simulink model "VehicleModel_V3"  (R2021b)
settings: Solver=FixedStepAuto  StartTime=0.0  StopTime=4000  FixedStep=Max_StepSize  RelTol=1e-3
InitFcn:
  | addpath('./Include')
  | Vehicle_Parameters
undefined symbols (not defined in the file): Airpressure, drag_coeff, front_area, Gravity, Incline, Ion, Irradiance, Lithium, NextCoordDistance, Temperature, Volume
libraries: spsPVArrayLib x10, spsSeriesRLCBranchLib x10, fl_lib x10, spsCurrentMeasurementLib x7, nesl_utility x6, sdl_lib x5, spsVoltageMeasurementLib x4, spsIGBTDiodeLib x3, spsPWMGeneratorDCDCLib x3, slpidlib x1, spsGroundLib x1, spsBatteryLib x1
settings Model: SimulationMode=accelerator  Creator=Zubim  LastModifiedBy=Zubim
settings SolverCC: MaxConsecutiveZCs=1  ZeroCrossAlgorithm=Adaptive
settings DataIOCC: SaveState=on
settings OptimizationCC: SimCompilerOptimization=on
settings DebuggingCC: StringTruncationChecking=none  IgnoredZcDiagnostic=none  MultiTaskCondExecSysMsg=none  MultiTaskRateTransMsg=warning  TasksWithSamePriorityMsg=none  SigSpecEnsureSampleTimeMsg=none  IntegerOverflowMsg=none  UnknownTsInhSupMsg=none  IntegerSaturationMsg=none
settings SFSimCC: SimCtrlC=off

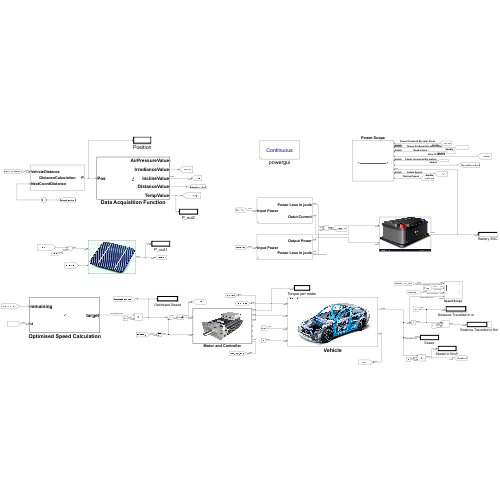
[thumbnail: Simulink's stored preview of the top-level diagram]
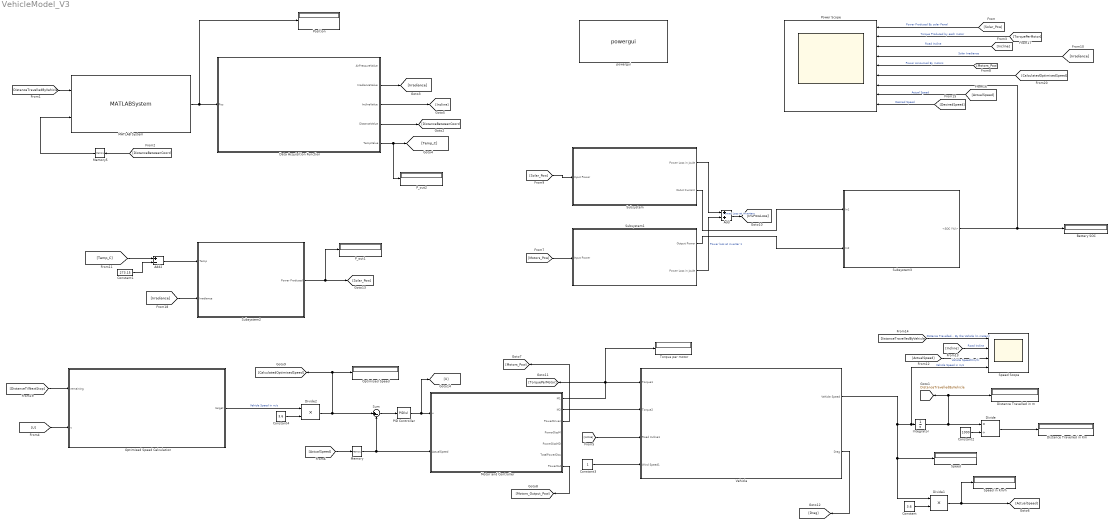
== system VehicleModel_V3 ==
  Add : Sum
  Add2 : Sum  Inputs=+-
  Battery SOC : Display
  Constant : Constant  Value=3.6
  Constant1 : Constant  Value=273.15
  Constant2 : Constant  Value=1000
  Constant3 : Constant
  Constant4 : Constant  Value=3.6
  Data Acquisition Function : MATLAB Function  TreatAsAtomicUnit=on
  Distance Travelled in Km : Display
  Distance Travelled in m : Display
  Divide : Product  Inputs=*/
  Divide1 : Product  Inputs=**
  Divide2 : Product  Inputs=**
  Integrator : Integrator
  MATLAB System : MATLABSystem  System=DistanceCalculation  SimulateUsing=Code generation
      mask Type: DistanceCalculation
      mask Display:
      | disp('DistanceCalculation');
      | port_label('input',1,'VehicleDistance');
      | port_label('input',2,'NextCoordDistance');
      | port_label('output',1,'P');
  Memory : Memory
  Memory5 : Memory  InheritSampleTime=on  LinearizeAsDelay=on
  Motor and Controller : MATLAB Function  TreatAsAtomicUnit=on
  Optimised Speed : Display
  Optimised Speed Calculation : MATLAB Function  TreatAsAtomicUnit=on
  PID Controller : slpidlib/PID Controller  Controller=PID  Form=Parallel  TimeDomain=Continuous-time  UseExternalTs=off  SampleTime=-1  IntegratorMethod=Forward Euler  FilterMethod=Forward Euler  ControllerParametersSource=internal  P=7.5E-1  I=15E-5  D=1.15E-1  UseFilter=on  N=1  TunerSelectOption=Transfer Function Based (PID Tuner App)  InitialConditionSource=internal  InitialConditionForIntegrator=0  InitialConditionForFilter=0  DifferentiatorICPrevScaledInput=0  ExternalReset=none  TrackingMode=off  Kt=1  LimitOutput=on  SatLimitsSource=internal  UpperSaturationLimit=1  LowerSaturationLimit=-0.2  LinearizeAsGain=on  AntiWindupMode=none  Kb=1  POutMin=[]  POutMax=[]  IOutMin=[]  IOutMax=[]  DOutMin=[]  DOutMax=[]  NOutMin=[]  NOutMax=[]  SumOutDataTypeStr=double  SumOutMin=[]  SumOutMax=[]  SaturationOutDataTypeStr=double  SaturationOutMin=[]  SaturationOutMax=[]  PParamMin=[]  PParamMax=[]  IParamMin=[]  IParamMax=[]  DParamMin=[]  DParamMax=[]  NParamMin=[]  NParamMax=[]  KbParamMin=[]  KbParamMax=[]  KtParamMin=[]  KtParamMax=[]  KbOutMin=[]  KbOutMax=[]  KtOutMin=[]  KtOutMax=[]  IntegratorOutMin=[]  IntegratorOutMax=[]  FilterOutMin=[]  FilterOutMax=[]  SumI1OutMin=[]  SumI1OutMax=[]  SumI2OutMin=[]  SumI2OutMax=[]  SumI3OutMin=[]  SumI3OutMax=[]  SumI4OutMin=[]  SumI4OutMax=[]  SumDOutMin=[]  SumDOutMax=[]  DifferentiatorOutMin=[]  DifferentiatorOutMax=[]  FilterDiffOutCoefMin=[]  FilterDiffOutCoefMax=[]  ReciprocalOutMin=[]  ReciprocalOutMax=[]  SumDenOutMin=[]  SumDenOutMax=[]  SumNumOutMin=[]  SumNumOutMax=[]  DivideOutMin=[]  DivideOutMax=[]  UdiffTsProdOutMin=[]  UdiffTsProdOutMax=[]  NTsProdOutMin=[]  NTsProdOutMax=[]  UintegralTsProdOutMin=[]  UintegralTsProdOutMax=[]  UngainTsProdOutMin=[]  UngainTsProdOutMax=[]  IntegratorContinuousStateAttributes=''  IntegratorStateMustResolveToSignalObject=off  IntegratorRTWStateStorageClass=Auto  FilterContinuousStateAttributes=''  FilterStateMustResolveToSignalObject=off  FilterRTWStateStorageClass=Auto  ParallelPVariant=InternalParameters  IdealPVariant=Disabled  IVariant=InternalParameters  DVariant=InternalParameters  IntegratorVariant=Continuous  SatVariant=Enabled  AWVariant=Passthrough  PCopyVariant=Disabled  TRVariant=Disabled  FdbkBlocksVariant=Forward  IdealPFdbkVariant=Disabled  SatFdbkVariant=Disabled  DerivativeFilterVariant=ContFilter  NVariant=InternalParameters  NCopyVariant=Disabled  FilterICVariant=InternalICsFilter  IntegratorICVariant=InternalICs  ExternalResetVariant=Disabled  TRSumVariant=Passthrough  SumFdbkVariant=Disabled  SumVariant=Sum_PID  TsampFilterVariant=InternalTs  TsampNgainVariant=Passthrough  TsampIntegralVariant=Passthrough  ExternalSaturationOutDataTypeStr=Inherit: Same as second input
  P_out1 : Display
  P_out2 : Display
  Position : Display
  Power Scope : Scope  NumInputPorts=9
  Speed : Display
  Speed Scope : Scope  NumInputPorts=4
  Speed in Km/h : Display
  Subsystem : Subsystem  mask{Inv_Efficiency=0.99}
      mask prompts: Inv_Efficiency "Efficiency (value between  0 and 1)"
  Subsystem1 : Subsystem  mask{Inv_Efficiency=0.95}
      mask prompts: Inv_Efficiency "Efficiency (value between  0 and 1)"
  Subsystem2 : Subsystem
      mask Display: image('D:\Vehicle Model\Images\Solar_cell.png'); % Use "Edit Image" on toolstrip to change.
  Subsystem3 : Subsystem
      mask Display: image('D:\Vehicle Model\Images\Battery.jpg'); % Use "Edit Image" on toolstrip to change.
  Sum : Sum  Inputs=|+-
  Torque per motor : Display
  Vehicle : Subsystem
      mask Display: image('D:\3rd Year\Group Project\Vehicle Model Matlab\Vehicle.jpg'); % Use "Edit Image" on toolstrip to change.
  powergui : spspowerguiLib/powergui  Priority=1  SimulationMode=Continuous  SampleTime=1  frequency=60  Iterations=50  frequencyindice=0  Pbase=100e6  ErrMax=1e-4  UnitsV=kV  UnitsW=MW  buscounter=0  FunctionMessages=off  echomessages=off  EnableUseOfTLC=off  CurrentSourceSwitches=off  DisableSnubberDevices=off  DisableRonSwitches=off  DisableVfSwitches=off  DisplayEquations=off  AutomaticDiscreteSolvers=off  SolverType=Tustin/Backward Euler (TBE)  Interpol=off  ExternalGateDelay=off  methode=off  Ts=100  x0status=blocks  SPID=on  SwTol=0  HookPort=off  NonlinearTolerance=1e-4  nMaxIteration=100  ContinueOnMaxIteration=off  RestoreLinks=warning  ResistiveCurrentMeasurement=off  Frange=[0:2:500]  Ylog=off  Xlog=on  ShowGrid=off  save=off  variable=ZData  structure=0  ZoomFFT=off  StartTime=0.0  cycles=1  DisplayStyle=1  fundamental=60  FreqAxis=off  MaxFrequency=1000  frequencyindicesteady=1  RmsSteady=1  display=off
  tag scope: DistanceTravelledByVehicle=global
  wires:
  Subsystem/1(" Power Loss in joule") -> Add/1
  Vehicle/1(Vehicle Speed) -> Speed Scope/4, Integrator/1, Speed/1, Divide1/1  "Vehicle Speed in m/s"
  [DistanceTravelledByVehicle] -> MATLAB System/1
  [DistanceBetweenCoord] -> Memory5/1
  Memory5/1 -> MATLAB System/2
  Constant2/1 -> Divide/2
  Divide/1 -> Distance Travelled in Km/1
  [Incline] -> Vehicle/3(Road Incline1)
  [Solar_Pow] -> Subsystem/1(Input Power)
  MATLAB System/1 -> Position/1, Data Acquisition Function/1(Pos)
  Data Acquisition Function/4(DistanceValue) -> [DistanceBetweenCoord]
  Data Acquisition Function/2(IrradianceValue) -> [Irradiance]
  Data Acquisition Function/5(TempValue) -> P_out2/1, [Temp_C]
  Data Acquisition Function/3(InclineValue) -> [Incline]
  Sum/1 -> PID Controller/1
  PID Controller/1 -> [U], Motor and Controller/1(u)
  [ActualSpeed] -> Memory/1
  [Motors_Pow] -> Power Scope/5  "Power consumed By motors"
  [Irradiance] -> Power Scope/4  "Solar Irradiance"
  Memory/1 -> Sum/2, Motor and Controller/2(ActualSpeed)
  Motor and Controller/2(M2) -> Vehicle/2(Torque2)
  Motor and Controller/1(M1) -> [TorquePerMotor], Torque per motor/1, Vehicle/1(Torque1)
  Constant3/1 -> Vehicle/4(Wind Speed1)
  Motor and Controller/3(PowerDriven) -> [Motors_Pow]
  Constant/1 -> Divide1/2
  Divide1/1 -> Speed in Km/h/1, [ActualSpeed]
  Integrator/1 -> [DistanceTravelledByVehicle], Distance Travelled in m/1, Divide/1
  [Incline] -> Power Scope/3  "Road Incline"
  [TorquePerMotor] -> Power Scope/2  "Torque Produced by each motor"
  [Motors_Pow] -> Subsystem1/1(Input Power)
  Subsystem1/2(" Power Loss in joule") -> Add/2  "Power loss at inverter 1"
  [ActualSpeed] -> Speed Scope/3  "Vehicle Speed(Km/h)"
  Motor and Controller/7(PowerOut) -> [Motors_Output_Pow]
  [Incline] -> Speed Scope/2  "Road Incline"
  [DistanceTravelledByVehicle] -> Speed Scope/1  "Distance Travelled By the Vehicle (in meters)"
  Add/1 -> [InvPowLoss]  "Power Loss at inverters"
  [DesiredSpeed] -> Power Scope/9  "Desired Speed"
  [Solar_Pow] -> Power Scope/1  "Power Produced By solar Penal"
  [ActualSpeed] -> Power Scope/8  "Actual Speed"
  Vehicle/2(Drag) -> [Drag]
  [Irradiance] -> Subsystem2/2(Irradiance)
  Add2/1 -> Subsystem2/1(Temp)
  Subsystem2/1(Power Produced) -> P_out1/1, [Solar_Pow]
  [Temp_C] -> Add2/1
  Constant1/1 -> Add2/2
  Subsystem3/1(<SOC (%)>) -> Battery SOC/1, Power Scope/7
  Subsystem/2(Outut Current) -> Subsystem3/1(In1)
  Subsystem1/1(Output Power) -> Subsystem3/2(In2)
  [U] -> Optimised Speed Calculation/2(u)
  [DistanceTilNextStop] -> Optimised Speed Calculation/1(remaining)
  Optimised Speed Calculation/1(target) -> Divide2/1  "Vehicle Speed in m/s"
  Divide2/1 -> Sum/1, Optimised Speed/1, [CalculatedOptimisedSpeed]
  Constant4/1 -> Divide2/2
  [CalculatedOptimisedSpeed] -> Power Scope/6

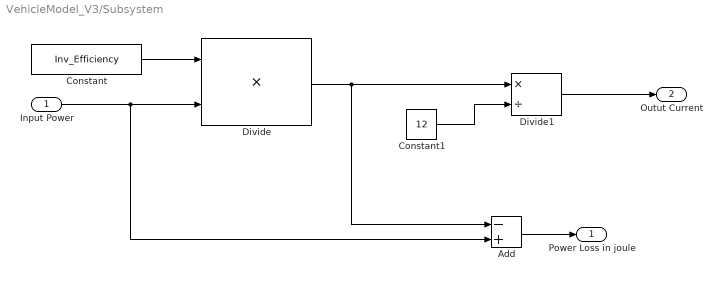
== system VehicleModel_V3/Subsystem ==
  Input Power : Inport
  Add : Sum  Inputs=-+
  Constant : Constant  Value=Inv_Efficiency
  Constant1 : Constant  Value=12
  Divide : Product  Inputs=**
  Divide1 : Product  Inputs=*/
  " Power Loss in joule" : Outport
  Outut Current : Outport  Port=2
  wires:
  Divide/1 -> Add/1, Divide1/1
  Input Power/1 -> Add/2, Divide/2
  Constant/1 -> Divide/1
  Add/1 -> " Power Loss in joule"/1
  Constant1/1 -> Divide1/2
  Divide1/1 -> Outut Current/1

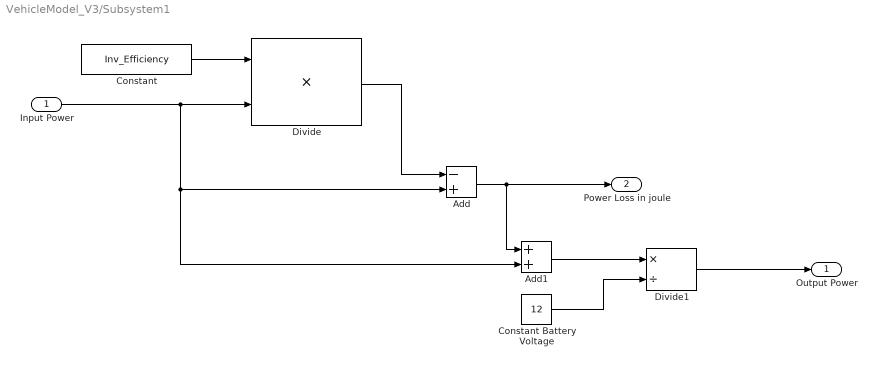
== system VehicleModel_V3/Subsystem1 ==
  Input Power : Inport
  Add : Sum  Inputs=-+
  Add1 : Sum
  Constant : Constant  Value=Inv_Efficiency
  Constant Battery Voltage : Constant  Value=12
  Divide : Product  Inputs=**
  Divide1 : Product  Inputs=*/
  Output Power : Outport
  " Power Loss in joule" : Outport  Port=2
  wires:
  Divide/1 -> Add/1
  Input Power/1 -> Add1/2, Add/2, Divide/2
  Constant/1 -> Divide/1
  Add/1 -> " Power Loss in joule"/1, Add1/1
  Constant Battery Voltage/1 -> Divide1/2
  Divide1/1 -> Output Power/1
  Add1/1 -> Divide1/1

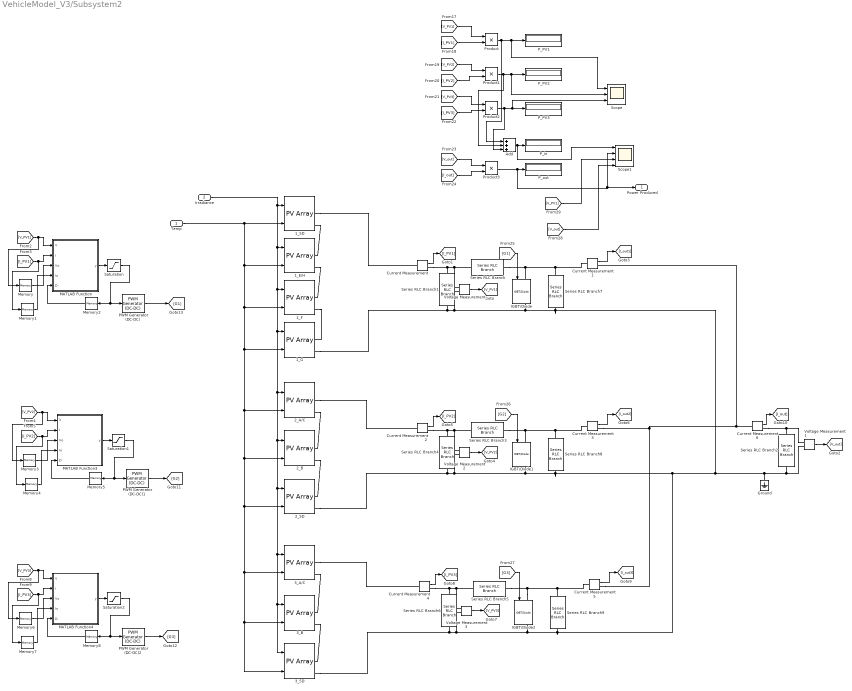
== system VehicleModel_V3/Subsystem2 ==
  Temp : Inport
  Irradiance : Inport  Port=2
  1_5D : spsPVArrayLib/PV Array  Npar=1  Nser=5  PlotType=one module @ 25 deg.C & specified irradiances  S_vec="[ 1000  500  100 ]"  Temp_C_vec="[ 45 25  ]"  ModuleName=User-defined  PlotWhenSelected=off  Pm=168.0338  Ncell=9  Voc=32.94  Isc=6.397  Vm=27.765  Im=6.052  beta_Voc_pc=-0.239  alpha_Isc_pc=0.0454  beta_Voc=-0.078727  alpha_Isc=0.0029042  IL=6.4028  I0=1.2931e-12  nI=4.8763  Rsh=312.183  Rs=0.25903  RobustModel=off  RobustCellTemperature=313.3991  BAL=on  Tc=1e-6  Tfilter=5e-5
  1_E/H : spsPVArrayLib/PV Array  Npar=1  Nser=2  PlotType=array @ 25 deg.C & specified irradiances  S_vec="[ 1000  500  100 ]"  Temp_C_vec="[ 45 25  ]"  ModuleName=User-defined  PlotWhenSelected=off  Pm=141.8952  Ncell=19  Voc=27.816  Isc=6.397  Vm=23.446  Im=6.052  beta_Voc_pc=-0.239  alpha_Isc_pc=0.0454  beta_Voc=-0.06648  alpha_Isc=0.0029042  IL=6.4023  I0=1.293e-12  nI=1.9505  Rsh=265.24  Rs=0.21875  RobustModel=off  RobustCellTemperature=313.3991  BAL=on  Tc=1e-6  Tfilter=5e-5
  1_F : spsPVArrayLib/PV Array  Npar=1  Nser=1  PlotType=array @ 25 deg.C & specified irradiances  S_vec="[ 1000  500  100 ]"  Temp_C_vec="[ 45 25  ]"  ModuleName=User-defined  PlotWhenSelected=off  Pm=52.2772  Ncell=14  Voc=10.248  Isc=6.397  Vm=8.638  Im=6.052  beta_Voc_pc=-0.239  alpha_Isc_pc=0.0454  beta_Voc=-0.024493  alpha_Isc=0.0029042  IL=6.4057  I0=1.3098e-12  nI=0.97569  Rsh=93.1389  Rs=0.080506  RobustModel=off  RobustCellTemperature=313.3991  BAL=on  Tc=1e-6  Tfilter=5e-5
  1_G : spsPVArrayLib/PV Array  Npar=1  Nser=1  PlotType=array @ 25 deg.C & specified irradiances  S_vec="[ 1000  500  100 ]"  Temp_C_vec="[ 45 25  ]"  ModuleName=User-defined  PlotWhenSelected=off  Pm=56.0113  Ncell=15  Voc=10.98  Isc=6.397  Vm=9.255  Im=6.052  beta_Voc_pc=-0.239  alpha_Isc_pc=0.0454  beta_Voc=-0.026242  alpha_Isc=0.0029042  IL=6.4023  I0=1.3098e-12  nI=0.97568  Rsh=104.8272  Rs=0.086285  RobustModel=off  RobustCellTemperature=313.3991  BAL=on  Tc=1e-6  Tfilter=5e-5
  2_5D : spsPVArrayLib/PV Array  Npar=1  Nser=5  PlotType=array @ 25 deg.C & specified irradiances  S_vec="[ 1000  500  100 ]"  Temp_C_vec="[ 45 25  ]"  ModuleName=User-defined  PlotWhenSelected=off  Pm=168.0338  Ncell=9  Voc=32.94  Isc=6.397  Vm=27.765  Im=6.052  beta_Voc_pc=-0.239  alpha_Isc_pc=0.0454  beta_Voc=-0.078727  alpha_Isc=0.0029042  IL=6.4028  I0=1.2931e-12  nI=4.8763  Rsh=312.183  Rs=0.25903  RobustModel=off  RobustCellTemperature=313.3991  BAL=on  Tc=1e-6  Tfilter=5e-5
  2_A/C : spsPVArrayLib/PV Array  Npar=1  Nser=2  PlotType=array @ 25 deg.C & specified irradiances  S_vec="[ 1000  500  100 ]"  Temp_C_vec="[ 45 25  ]"  ModuleName=User-defined  PlotWhenSelected=off  Pm=179.236  Ncell=24  Voc=35.136  Isc=6.397  Vm=29.616  Im=6.052  beta_Voc_pc=-0.239  alpha_Isc_pc=0.0454  beta_Voc=-0.083975  alpha_Isc=0.0029042  IL=6.4082  I0=1.3104e-12  nI=1.9514  Rsh=314.3068  Rs=0.27595  RobustModel=off  RobustCellTemperature=313.3991  BAL=on  Tc=1e-6  Tfilter=5e-5
  2_B : spsPVArrayLib/PV Array  Npar=1  Nser=1  PlotType=array @ 25 deg.C & specified irradiances  S_vec="[ 1000  500  100 ]"  Temp_C_vec="[ 45 25  ]"  ModuleName=User-defined  PlotWhenSelected=off  Pm=44.809  Ncell=12  Voc=8.784  Isc=6.397  Vm=7.404  Im=6.052  beta_Voc_pc=-0.239  alpha_Isc_pc=0.0454  beta_Voc=-0.020994  alpha_Isc=0.0029042  IL=6.4257  I0=1.3106e-12  nI=0.97584  Rsh=56.9513  Rs=0.068881  RobustModel=off  RobustCellTemperature=313.3991  BAL=on  Tc=1e-6  Tfilter=5e-5
  3_5D : spsPVArrayLib/PV Array  Npar=1  Nser=5  PlotType=array @ 25 deg.C & specified irradiances  S_vec="[ 1000  500  100 ]"  Temp_C_vec="[ 45 25  ]"  ModuleName=User-defined  PlotWhenSelected=off  Pm=168.0338  Ncell=9  Voc=32.94  Isc=6.397  Vm=27.765  Im=6.052  beta_Voc_pc=-0.239  alpha_Isc_pc=0.0454  beta_Voc=-0.078727  alpha_Isc=0.0029042  IL=6.4028  I0=1.2931e-12  nI=4.8763  Rsh=312.183  Rs=0.25903  RobustModel=off  RobustCellTemperature=313.3991  BAL=on  Tc=1e-6  Tfilter=5e-5
  3_A/C : spsPVArrayLib/PV Array  Npar=1  Nser=2  PlotType=array @ 25 deg.C & specified irradiances  S_vec="[ 1000  500  100 ]"  Temp_C_vec="[ 45 25  ]"  ModuleName=User-defined  PlotWhenSelected=off  Pm=179.236  Ncell=24  Voc=35.136  Isc=6.397  Vm=29.616  Im=6.052  beta_Voc_pc=-0.239  alpha_Isc_pc=0.0454  beta_Voc=-0.083975  alpha_Isc=0.0029042  IL=6.4082  I0=1.3104e-12  nI=1.9514  Rsh=314.3068  Rs=0.27595  RobustModel=off  RobustCellTemperature=313.3991  BAL=on  Tc=1e-6  Tfilter=5e-5
  3_B : spsPVArrayLib/PV Array  Npar=1  Nser=1  PlotType=array @ 25 deg.C & specified irradiances  S_vec="[ 1000  500  100 ]"  Temp_C_vec="[ 45 25  ]"  ModuleName=User-defined  PlotWhenSelected=off  Pm=44.809  Ncell=12  Voc=8.784  Isc=6.397  Vm=7.404  Im=6.052  beta_Voc_pc=-0.239  alpha_Isc_pc=0.0454  beta_Voc=-0.020994  alpha_Isc=0.0029042  IL=6.4257  I0=1.3106e-12  nI=0.97584  Rsh=56.9513  Rs=0.068881  RobustModel=off  RobustCellTemperature=313.3991  BAL=on  Tc=1e-6  Tfilter=5e-5
  Add : Sum  Inputs=+++
  Current Measurement{,1..6} (7 alike) : spsCurrentMeasurementLib/Current Measurement  PhasorSimulation=off  OutputType=Complex  PSBequivalent=0
  Ground : spsGroundLib/Ground  LConnTagsString=a
  IGBT/Diode : spsIGBTDiodeLib/IGBT//Diode  Ron=1e-3  Rs=1e5  Cs=inf  Measurements=on
  IGBT/Diode1 : spsIGBTDiodeLib/IGBT//Diode  Ron=1e-3  Rs=1e5  Cs=inf  Measurements=on
  IGBT/Diode2 : spsIGBTDiodeLib/IGBT//Diode  Ron=1e-3  Rs=1e5  Cs=inf  Measurements=on
  MATLAB Function : MATLAB Function  TreatAsAtomicUnit=on
  MATLAB Function3 : MATLAB Function  TreatAsAtomicUnit=on
  MATLAB Function4 : MATLAB Function  TreatAsAtomicUnit=on
  Memory{,1..8} (9 alike) : Memory
  PWM Generator (DC-DC) : spsPWMGeneratorDCDCLib/PWM Generator (DC-DC)  Fsw=5000  Ts=0
  PWM Generator (DC-DC)1 : spsPWMGeneratorDCDCLib/PWM Generator (DC-DC)  Fsw=5000  Ts=0
  PWM Generator (DC-DC)2 : spsPWMGeneratorDCDCLib/PWM Generator (DC-DC)  Fsw=5000  Ts=0
  P_PV1 : Display
  P_PV2 : Display
  P_PV3 : Display
  P_in : Display
  P_out : Display
  Product{,1..3} (4 alike) : Product
  Saturation : Saturate  LowerLimit=0
  Saturation1 : Saturate  LowerLimit=0
  Saturation2 : Saturate  LowerLimit=0
  Scope : Scope  NumInputPorts=3
  Scope1 : Scope  NumInputPorts=4
  Series RLC Branch : spsSeriesRLCBranchLib/Series RLC Branch  LConnTagsString=__new0  RConnTagsString=__new0  BranchType=RL  Resistance=0.0005  Inductance=0.055  SetiL0=off  InitialCurrent=0  Capacitance=1e-6  Setx0=off  InitialVoltage=0  Measurements=None
  Series RLC Branch1 : spsSeriesRLCBranchLib/Series RLC Branch  LConnTagsString=__new0  RConnTagsString=__new0  BranchType=C  Resistance=0.0005  Inductance=0.055  SetiL0=off  InitialCurrent=0  Capacitance=10e-6  Setx0=off  InitialVoltage=0  Measurements=None
  Series RLC Branch2 : spsSeriesRLCBranchLib/Series RLC Branch  LConnTagsString=__new0  RConnTagsString=__new0  BranchType=R  Resistance=30  Inductance=0.055  SetiL0=off  InitialCurrent=0  Capacitance=1e-6  Setx0=off  InitialVoltage=0  Measurements=None
  Series RLC Branch3 : spsSeriesRLCBranchLib/Series RLC Branch  LConnTagsString=__new0  RConnTagsString=__new0  BranchType=RL  Resistance=0.0005  Inductance=0.055  SetiL0=off  InitialCurrent=0  Capacitance=1e-6  Setx0=off  InitialVoltage=0  Measurements=None
  Series RLC Branch4 : spsSeriesRLCBranchLib/Series RLC Branch  LConnTagsString=__new0  RConnTagsString=__new0  BranchType=C  Resistance=0.0005  Inductance=0.055  SetiL0=off  InitialCurrent=0  Capacitance=10e-6  Setx0=off  InitialVoltage=0  Measurements=None
  Series RLC Branch5 : spsSeriesRLCBranchLib/Series RLC Branch  LConnTagsString=__new0  RConnTagsString=__new0  BranchType=RL  Resistance=0.0005  Inductance=0.055  SetiL0=off  InitialCurrent=0  Capacitance=1e-6  Setx0=off  InitialVoltage=0  Measurements=None
  Series RLC Branch6 : spsSeriesRLCBranchLib/Series RLC Branch  LConnTagsString=__new0  RConnTagsString=__new0  BranchType=C  Resistance=0.0005  Inductance=0.055  SetiL0=off  InitialCurrent=0  Capacitance=10e-6  Setx0=off  InitialVoltage=0  Measurements=None
  Series RLC Branch7 : spsSeriesRLCBranchLib/Series RLC Branch  LConnTagsString=__new0  RConnTagsString=__new0  BranchType=C  Resistance=0.0005  Inductance=0.055  SetiL0=off  InitialCurrent=0  Capacitance=1e-6  Setx0=off  InitialVoltage=0  Measurements=None
  Series RLC Branch8 : spsSeriesRLCBranchLib/Series RLC Branch  LConnTagsString=__new0  RConnTagsString=__new0  BranchType=C  Resistance=0.0005  Inductance=0.055  SetiL0=off  InitialCurrent=0  Capacitance=1e-6  Setx0=off  InitialVoltage=0  Measurements=None
  Series RLC Branch9 : spsSeriesRLCBranchLib/Series RLC Branch  LConnTagsString=__new0  RConnTagsString=__new0  BranchType=C  Resistance=0.0005  Inductance=0.055  SetiL0=off  InitialCurrent=0  Capacitance=1e-6  Setx0=off  InitialVoltage=0  Measurements=None
  Voltage Measurement{,1..3} (4 alike) : spsVoltageMeasurementLib/Voltage Measurement  PhasorSimulation=off  OutputType=Complex  PSBequivalent=0
  Power Produced : Outport
  wires:
  Voltage Measurement3/1 -> [V_PV3]
  [I_PV1] -> Memory1/1, MATLAB Function/2(I)
  PWM Generator (DC-DC)/1 -> [G1]
  Current Measurement5/1 -> [I_out3]
  Memory1/1 -> MATLAB Function/4(Io)
  Current Measurement1/1 -> [I_out1]
  Product3/1 -> Power Produced/1, Scope1/2, P_out/1
  Saturation/1 -> PWM Generator (DC-DC)/1, Memory2/1
  Voltage Measurement/1 -> [V_PV1]
  Current Measurement/1 -> [I_PV1]
  [V_PV1] -> Memory/1, MATLAB Function/1(V)
  Current Measurement4/1 -> [I_PV3]
  Memory/1 -> MATLAB Function/3(Vo)
  Saturation2/1 -> PWM Generator (DC-DC)2/1, Memory8/1
  [G1] -> IGBT/Diode/1
  [I_PV2] -> Memory4/1, MATLAB Function3/2(I)
  MATLAB Function/1(y) -> Saturation/1
  [V_out] -> Product3/1
  [V_PV2] -> Memory3/1, MATLAB Function3/1(V)
  MATLAB Function3/1(y) -> Saturation1/1
  Current Measurement2/1 -> [I_PV2]
  [V_PV1] -> Product/1
  Memory3/1 -> MATLAB Function3/3(Vo)
  Product1/1 -> Scope/2, P_PV2/1, Add/2
  Saturation1/1 -> PWM Generator (DC-DC)1/1, Memory5/1
  Memory2/1 -> MATLAB Function/5(D)
  MATLAB Function4/1(y) -> Saturation2/1
  [I_PV1] -> Product/2
  Irradiance/1 -> 2_5D/1, 3_B/1, 3_5D/1, 3_A/C/1, 2_B/1, 2_A/C/1, 1_G/1, 1_F/1, 1_E/H/1, 1_5D/1
  Memory7/1 -> MATLAB Function4/4(Io)
  Current Measurement6/1 -> [I_out]
  Temp/1 -> 1_5D/2, 1_E/H/2, 1_F/2, 2_5D/2, 3_B/2, 3_5D/2, 3_A/C/2, 2_B/2, 2_A/C/2, 1_G/2
  Voltage Measurement1/1 -> [V_out]
  Add/1 -> Scope1/1, P_in/1
  Product/1 -> Add/1, Scope/1, P_PV1/1
  [I_PV3] -> Memory7/1, MATLAB Function4/2(I)
  [V_out] -> Scope1/4
  Memory4/1 -> MATLAB Function3/4(Io)
  Memory8/1 -> MATLAB Function4/5(D)
  [G2] -> IGBT/Diode1/1
  [V_PV3] -> Product2/1
  PWM Generator (DC-DC)2/1 -> [G3]
  [I_PV2] -> Product1/2
  PWM Generator (DC-DC)1/1 -> [G2]
  [I_PV3] -> Product2/2
  Memory5/1 -> MATLAB Function3/5(D)
  Current Measurement3/1 -> [I_out2]
  Product2/1 -> Scope/3, P_PV3/1, Add/3
  [V_PV3] -> Memory6/1, MATLAB Function4/1(V)
  [G3] -> IGBT/Diode2/1
  [I_out] -> Product3/2
  Voltage Measurement2/1 -> [V_PV2]
  [V_PV2] -> Product1/1
  Memory6/1 -> MATLAB Function4/3(Vo)
  [V_PV1] -> Scope1/3
  connections:
  IGBT/Diode2/LConn1 -- Series RLC Branch5/RConn1 -- Series RLC Branch9/LConn1 -- Current Measurement5/LConn1
  Voltage Measurement2/LConn1 -- Series RLC Branch3/LConn1 -- Series RLC Branch4/LConn1 -- Current Measurement2/RConn1
  Current Measurement6/RConn1 -- Series RLC Branch2/RConn1 -- Voltage Measurement1/LConn1
  Series RLC Branch7/LConn1 -- Current Measurement1/LConn1 -- Series RLC Branch/RConn1 -- IGBT/Diode/LConn1
  Voltage Measurement/LConn2 -- Series RLC Branch1/RConn1 -- 1_G/RConn2 -- IGBT/Diode/RConn1 -- Series RLC Branch7/RConn1 -- Series RLC Branch8/RConn1 -- IGBT/Diode1/RConn1 -- 2_5D/RConn2 -- Series RLC Branch4/RConn1 -- Voltage Measurement2/LConn2 -- Series RLC Branch9/RConn1 -- IGBT/Diode2/RConn1 -- 3_5D/RConn2 -- Series RLC Branch6/RConn1 -- Voltage Measurement3/LConn2 -- Ground/LConn1 -- Series RLC Branch2/LConn1 -- Voltage Measurement1/LConn2
  Current Measurement3/RConn1 -- Current Measurement6/LConn1 -- Current Measurement1/RConn1 -- Current Measurement5/RConn1
  Current Measurement3/LConn1 -- Series RLC Branch8/LConn1 -- Series RLC Branch3/RConn1 -- IGBT/Diode1/LConn1
  3_A/C/RConn2 -- 3_B/RConn1
  Voltage Measurement3/LConn1 -- Series RLC Branch5/LConn1 -- Series RLC Branch6/LConn1 -- Current Measurement4/RConn1
  Series RLC Branch1/LConn1 -- Current Measurement/RConn1 -- Series RLC Branch/LConn1 -- Voltage Measurement/LConn1
  3_A/C/RConn1 -- Current Measurement4/LConn1
  1_F/RConn2 -- 1_G/RConn1
  1_E/H/RConn2 -- 1_F/RConn1
  1_5D/RConn2 -- 1_E/H/RConn1
  2_B/RConn2 -- 2_5D/RConn1
  2_A/C/RConn1 -- Current Measurement2/LConn1
  3_B/RConn2 -- 3_5D/RConn1
  2_A/C/RConn2 -- 2_B/RConn1
  1_5D/RConn1 -- Current Measurement/LConn1

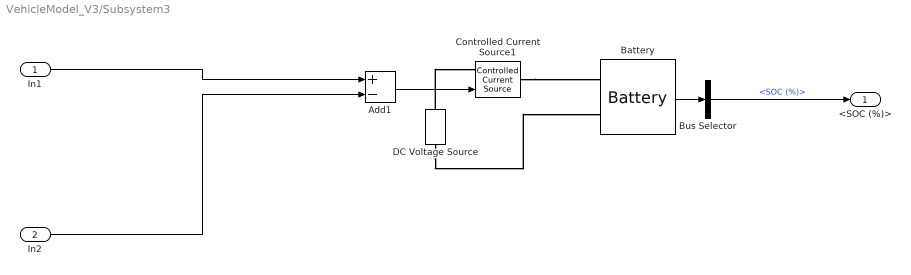
== system VehicleModel_V3/Subsystem3 ==
  In1 : Inport
  In2 : Inport  Port=2
  Add1 : Sum  Inputs=+-
  Battery : spsBatteryLib/Battery  BatType=Lithium-Ion  ShowTempParam=off  ThermalPreset=no  ShowAgeParam=off  NomV=12  NomQ=200  SOC=50  Batt_Tr=30  PresetModel=on  MaxQ=200  MinV=9  FullV=13.9678  Dis_rate=86.9565  R=0.0006  Normal_OP=180.8696  expZone="[12.9646      9.82609]"  current=[6.5 13 32.5]  Units=Time  Tci=20  NomT=20  T2=-30  MaxQ2=4.8  FullV2=7.1  Normal_OP2=5.655  expZone2="[6.58           1]"  Rca=0.6  ti=2000  Dp=0  Neq0=0  Tsim=1e6  Ta1=25  Qeol=5.4*0.9  Reol=0.013333*1.2  Char_age=[2.3478, 3]  Dis_age=[2.3478, 10]  N1=1500  N2=10500  N3=1000  N4=1400  Ta2=45  N5=950
  Bus Selector : BusSelector  OutputSignals=SOC (%)
  Controlled Current Source1 : spsControlledCurrentSourceLib/Controlled Current Source  Initialize=on  Source_Type=AC  Amplitude=0  Phase=0  Frequency=0  Measurements=None
  DC Voltage Source : spsDCVoltageSourceLib/DC Voltage Source  Amplitude=12  Measurements=None
  <SOC (%)> : Outport
  wires:
  Bus Selector/1 -> <SOC (%)>/1  "<SOC (%)>"
  Add1/1 -> Controlled Current Source1/1
  In1/1 -> Add1/1
  Battery/1 -> Bus Selector/1
  In2/1 -> Add1/2
  connections:
  Controlled Current Source1/RConn1 -- Battery/LConn1
  DC Voltage Source/RConn1 -- Controlled Current Source1/LConn1
  DC Voltage Source/LConn1 -- Battery/LConn2

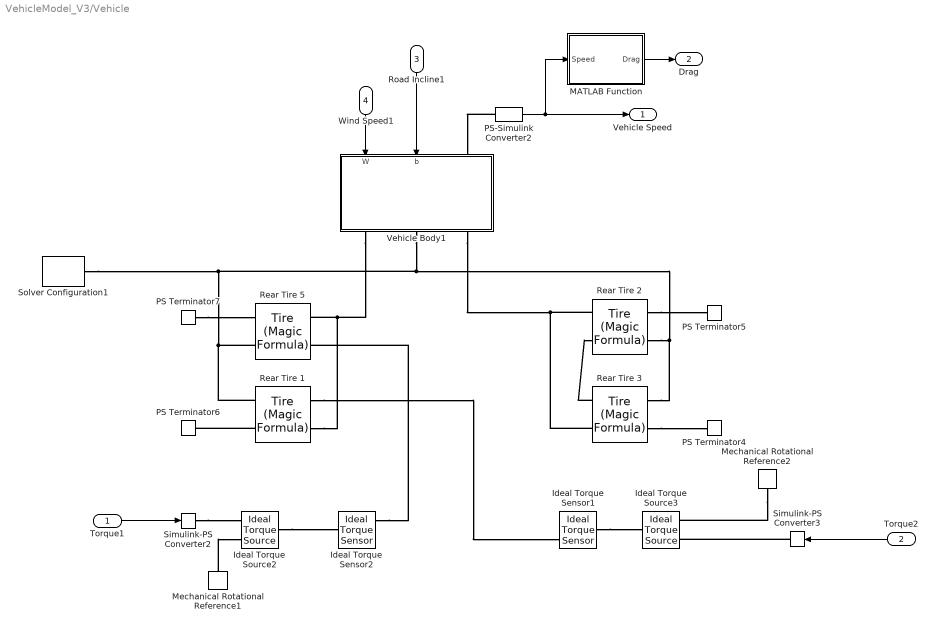
== system VehicleModel_V3/Vehicle ==
  Torque1 : Inport
  Torque2 : Inport  Port=2
  Road Incline1 : Inport  Port=3
  Wind Speed1 : Inport  Port=4
  Ideal Torque Sensor1 : fl_lib/Mechanical/Mechanical Sensors/Ideal Torque Sensor
  Ideal Torque Sensor2 : fl_lib/Mechanical/Mechanical Sensors/Ideal Torque Sensor
  Ideal Torque Source2 : fl_lib/Mechanical/Mechanical Sources/Ideal Torque Source
  Ideal Torque Source3 : fl_lib/Mechanical/Mechanical Sources/Ideal Torque Source
  MATLAB Function : MATLAB Function  TreatAsAtomicUnit=on
  Mechanical Rotational Reference1 : fl_lib/Mechanical/Rotational Elements/Mechanical Rotational Reference
  Mechanical Rotational Reference2 : fl_lib/Mechanical/Rotational Elements/Mechanical Rotational Reference
  PS Terminator{4..7} (4 alike) : fl_lib/Physical Signals/Sinks/PS Terminator
  PS-Simulink Converter2 : nesl_utility/PS-Simulink Converter  PhysicalDomain=network_engine_domain  SubClassName=ps_output  LeftPortType=input  RightPortType=output  PseudoPeriodic=off  Frequencies=[]  Unit=m/s  AffineConversion=off
      settings: SourceProductBaseCode=PW,SS
  Rear Tire {1..3,5} (4 alike) : sdl_lib/Tires & Vehicles/Tire (Magic Formula)  parameterization=sdl.enum.magic_tire_model.peak  F_z1=3000 N  F_x1=3500 N  kappa1=10  B_m=tire_b  C_m=tire_c  D_m=tire_d  E_m=tire_e  fz0=4000 N  p_Cx=1.685  p_Dx=[1.21, -.037]  p_Ex=[.344, .095, -.02, 0]  p_Kx=[21.51, -.163, .245]  p_Hx=[-.002, .002]  p_Vx=[0, 0]  r_e=Rolling_Radius m  model_compliance=sdl.enum.compliance.off  stiffness=1e6 N/m  damping=1000 N/(m/s)  model_inertia=sdl.enum.model_inertia.on  inertia=tire_inertia kg*m^2  initial_velocity=0 rad/s  model_resistance=simscape.enum.onoff.on  resistance_model=sdl.enum.rollingResistanceParameterization.constant  coeff=roll_resist  p_tire=250e3 Pa  alpha=-0.003  beta=0.97  coeff_a=84e-4  coeff_b=6.2e-4 s/m  coeff_c=1.6e-4 s^2/m^2  v_thr=0.001 m/s  v_tr_thr=0.1 m/s
  Simulink-PS Converter2 : nesl_utility/Simulink-PS Converter  PhysicalDomain=network_engine_domain  SubClassName=ps_input  LeftPortType=input  RightPortType=output  PseudoPeriodic=off  Frequencies=[]  NoiseDistribution=none  NoiseParameters=[]  Unit=N*m  AffineConversion=on  FilteringAndDerivatives=provide  SimscapeFilterOrder=1  InputFilterTimeConstant=0.001  UdotUserProvided=0
      settings: SourceProductBaseCode=PW,SS
  Simulink-PS Converter3 : nesl_utility/Simulink-PS Converter  PhysicalDomain=network_engine_domain  SubClassName=ps_input  LeftPortType=input  RightPortType=output  PseudoPeriodic=off  Frequencies=[]  NoiseDistribution=none  NoiseParameters=[]  Unit=N*m  AffineConversion=on  FilteringAndDerivatives=provide  SimscapeFilterOrder=1  InputFilterTimeConstant=0.001  UdotUserProvided=0
      settings: SourceProductBaseCode=PW,SS
  Solver Configuration1 : nesl_utility/Solver Configuration  PhysicalDomain=network_engine_domain  SubClassName=solver  LeftPortType=input  RightPortType=generic  Tones=[]  Harmonics=[]  SimulateNoise=off  Profile=off  UseLocalSampling=off  EnableSwitchedLinearOptims=on  FrequencyDomain=off  UseCCode=off  RelTol=0.001  AbsTol=1e-06  MinStep=1e-09  ToWorkspace=off  RevertToSquareIcSolve=off  NumHomotopyIterations=100  PhasorMode=off  PhasorModeNumHarmonics=1  DoDC=off  ResidualTolerance=1e-09  UseLocalSolver=off  LocalSolverChoice=NE_BACKWARD_EULER_ADVANCER  LocalSolverSampleTime=0.001  DoFixedCost=off  MaxNonlinIter=3  MaxModeIter=2  ComputeImpulses=off  ImpulseIterations=2  LinearAlgebra=auto  EquationFormulation=NE_TIME_EF  DelaysMemoryBudget=1024  AutomaticFiltering=on  FilteringTimeConstant=0.001  PartitionStorageMethod=AS_NEEDED  PartitionMemoryBudget=1024  PartitionMethod=ROBUST
      settings: SourceProductBaseCode=PW,SS
  Vehicle Body1 : Subsystem
      mask Display:
      | color('white')
      | plot(-120,-70); plot(120,40);
      | color('black')
      | plot(sin(0:0.1:6*pi)*15-70,cos(0:0.1:6*pi)*15-30);
      | plot(sin(0:0.1:6*pi)*15+70,cos(0:0.1:6*pi)*15-30);
      | plot([-88 -95 -99 -99 -95 -75 -65 -50 -46 10 30 34 80 85 90 93 95 93 90 88],[-30 -28 -23 -5 0 5 10 20 21 21 0 -2 -7 -9 -13 -17 -25 -28 -30 -30])
      | plot([-88 -95 -99 -99 -95 -75 -65 -50 -46 10 30 34 80 85 90 93 95 93 90 88],[-30 -28 -23 -5 0 5 10 20 21 21 0 -2 -7 -9 -13 -17 -25 -28 -30 -30]-1)
      | plot([-88 -95 -99 -99 -95 -75 -65 -50 -46 10 30 34 80 85 90 93 95 93 90 88]+1,[-30 -28 -23 -5 0 5 10 20 21 21 0 -2 -7 -9 -13 -17 -25 -28 -30 -30])
      | plot([-50 50],[-30 -30])
  Vehicle Speed : Outport
  Drag : Outport  Port=2
  wires:
  Torque2/1 -> Simulink-PS Converter3/1
  Torque1/1 -> Simulink-PS Converter2/1
  PS-Simulink Converter2/1 -> MATLAB Function/1(Speed), Vehicle Speed/1
  Road Incline1/1 -> Vehicle Body1/2(b)
  Wind Speed1/1 -> Vehicle Body1/1(W)
  MATLAB Function/1(Drag) -> Drag/1
  connections:
  Vehicle Body1/RConn2 -- Solver Configuration1/RConn1 -- Rear Tire 1/RConn2 -- Rear Tire 5/RConn2 -- Rear Tire 3/RConn2 -- Rear Tire 2/RConn2
  Rear Tire 5/LConn1 -- Rear Tire 1/LConn1 -- Vehicle Body1/RConn1
  Vehicle Body1/RConn3 -- Rear Tire 3/LConn1 -- Rear Tire 2/LConn1
  Rear Tire 2/RConn1 -- PS Terminator5/LConn1
  Rear Tire 3/RConn1 -- PS Terminator4/LConn1
  Mechanical Rotational Reference1/LConn1 -- Ideal Torque Source2/RConn2
  Mechanical Rotational Reference2/LConn1 -- Ideal Torque Source3/RConn2
  Rear Tire 1/LConn2 -- Ideal Torque Sensor1/RConn1
  PS Terminator7/LConn1 -- Rear Tire 5/RConn1
  Rear Tire 1/RConn1 -- PS Terminator6/LConn1
  Simulink-PS Converter3/RConn1 -- Ideal Torque Source3/RConn1
  Simulink-PS Converter2/RConn1 -- Ideal Torque Source2/RConn1
  PS-Simulink Converter2/LConn1 -- Vehicle Body1/LConn1
  Ideal Torque Sensor2/RConn1 -- Rear Tire 5/LConn2
  Ideal Torque Sensor1/LConn1 -- Ideal Torque Source3/LConn1
  Ideal Torque Source2/LConn1 -- Ideal Torque Sensor2/LConn1
  Rear Tire 3/LConn2 -- Rear Tire 2/LConn2

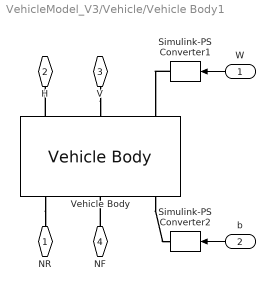
== system VehicleModel_V3/Vehicle/Vehicle Body1 ==
  W : Inport
  b : Inport  Port=2
  Simulink-PS Converter1 : nesl_utility/Simulink-PS Converter  PhysicalDomain=network_engine_domain  SubClassName=ps_input  LeftPortType=input  RightPortType=output  PseudoPeriodic=off  Frequencies=[]  NoiseDistribution=none  NoiseParameters=[]  Unit=m/s  AffineConversion=off  FilteringAndDerivatives=zero  SimscapeFilterOrder=1  InputFilterTimeConstant=.001  UdotUserProvided=1
      settings: SourceProductBaseCode=PW,SS
  Simulink-PS Converter2 : nesl_utility/Simulink-PS Converter  PhysicalDomain=network_engine_domain  SubClassName=ps_input  LeftPortType=input  RightPortType=output  PseudoPeriodic=off  Frequencies=[]  NoiseDistribution=none  NoiseParameters=[]  Unit=deg  AffineConversion=off  FilteringAndDerivatives=zero  SimscapeFilterOrder=1  InputFilterTimeConstant=Max_StepSize  UdotUserProvided=1
      settings: SourceProductBaseCode=PW,SS
  Vehicle Body : sdl_lib/Tires & Vehicles/Vehicle Body  mass=TotalVehicleMass kg  n_w=2  x_f=front_axle m  x_r=rear_axle m  y_c=CG_height m  mass_var=simscape.enum.onoff.off  g=Gravity m/s^2  liftoff_warning=simscape.enum.onoff.off  area=front_area m^2  Cd=drag_coeff  rho=Air_density kg/m^3  model_pitch=simscape.enum.onoff.off  inertia=4000 kg*m^2  suspension_model=sdl.enum.linearTLU.linear  k_f=1e4 N/m  b_f=1e4 N/(m/s)  k_r=1e4 N/m  b_r=1e4 N/(m/s)  k_f_TLU=[-2000, -1000, 0, 1000, 2000] N  x_f_TLU=[-.4, -.2, 0, .2, .4] m  b_f_TLU=[-200, -100, 0, 100, 200] N  v_f_TLU=[-4, -2, 0, 2, 4] m/s  k_r_TLU=[-2000, -1000, 0, 1000, 2000] N  x_r_TLU=[-.4, -.2, 0, .2, .4] m  b_r_TLU=[-200, -100, 0, 100, 200] N  v_r_TLU=[-4, -2, 0, 2, 4] m/s  interp_method=simscape.enum.interpolation.linear  extrap_method=simscape.enum.extrapolation.linear  model_hardstop=simscape.enum.onoff.off  upper_bound_f=.25 m  lower_bound_f=-.25 m  stop_k_f=1e6 N/m  stop_b_f=150 N/(m/s)  upper_bound_r=.25 m  lower_bound_r=-.25 m  stop_k_r=1e6 N/m  stop_b_r=150 N/(m/s)  initial_pitch=0 rad  initial_pitch_rate=0 rad/s  v_specify=on  v_priority=High  v=0 m/s  v_nominal_specify=off  v_nominal_unit=m/s  v_nominal_value=1
  NR : PMIOPort  Side=Right
  H : PMIOPort  Port=2  Side=Right
  V : PMIOPort  Port=3  Side=Left
  NF : PMIOPort  Port=4  Side=Right
  wires:
  W/1 -> Simulink-PS Converter1/1
  b/1 -> Simulink-PS Converter2/1
  connections:
  Simulink-PS Converter1/RConn1 -- Vehicle Body/LConn3
  Vehicle Body/LConn1 -- H/RConn1
  Vehicle Body/RConn3 -- Simulink-PS Converter2/RConn1
  NF/RConn1 -- Vehicle Body/RConn2
  V/RConn1 -- Vehicle Body/LConn2
  Vehicle Body/RConn1 -- NR/RConn1

== matlab function VehicleModel_V3/Data Acquisition Function ==
  data: Pos input; AirPressureValue output; Temperature parameter; Airpressure parameter; Irradiance parameter; Incline parameter; NextCoordDistance parameter; IrradianceValue output; InclineValue output; DistanceValue output; TempValue output
function [AirPressureValue,IrradianceValue,InclineValue,DistanceValue,TempValue] = fcn(Pos, Temperature, ...
    Airpressure, Irradiance, Incline, NextCoordDistance)

    AirPressureValue = Airpressure(Pos);
    IrradianceValue = Irradiance(Pos);
    InclineValue = Incline(Pos);
    DistanceValue = NextCoordDistance(Pos);
    TempValue = Temperature(Pos);
end

== matlab function VehicleModel_V3/Motor and Controller ==
  data: u input; M1 output; M2 output; PowerDriven output; PowerDissM output; ActualSpeed input; PowerDissMD output; TotalPowerDiss output; PowerOut output
% -------------------------- Function u --------------------------- %
%
% This Function calculates the percentage of torque demand for the 
% motors based on the difference between actual speed and desired
% speed using a PID controller.
%
% This function also calcualtes the total power loss due to 
% efficiencies as well as the power driven and outputted by the motors
%
% Authors: Robbie Walker
%
% --------------------- End of Description ------------------------ %


% -------------------------------------------------------------------------------------------- %
function [M1,M2,PowerDriven,PowerDissM,PowerDissMD,TotalPowerDiss,PowerOut] = fcn(u,ActualSpeed)
% -------------------------------------------------------------------------------------------- %


% ----------------- Function arguments ------------------ %
%
% M1 = M2 = Motor Torque (front and back)
% PowerDriven = Power driven to each motor
% PowerDissM = Power dissipated in the BLDC Motor
% PowerDissMD = Power dissipated in the motor drive (seperate to the motor)
% TotalPowerDiss = Total power dissipated in both the Motor and Motor Drive
% PowerOut = Actual power output from motors after losses
%
% ------------------------------------------------------- %


% -------- Function Variables ---------%

% Motor Parameters
MotorEfficiency = 98.3;  % percent
MaximumSpeed = 157;      % Rad/s
PeakTorque = 80;         %Nm
PeakContinuousTorque = 42;      %Nm
MinimumDriveEfficiency = 94 ;     % percent

% Wheel Parameters
MotorDiameter = 0.38;        % meters
TyreRimDiameter = 0.0762;    % meters

% -------------------------------------%


% ---------------- Calculations -----------------%

% Torque Driven to Motors
MotorTorque = PeakTorque * u;
M1 = MotorTorque;
M2 = MotorTorque;

% Total Diameter of Wheel
WheelDiameter = MotorDiameter+TyreRimDiameter;

% Speed
% m/s
MSSpeed = ActualSpeed/3.6;
% RPM
RPMSpeed = 9.55 * (MSSpeed/(WheelDiameter/2));
% rad/s
WSpeed = (RPMSpeed/60) * (2*3.14159);

% Motor Drive Efficiency at Motor Torque
DriveEfficiency = MinimumDriveEfficiency + (WSpeed*0.1);

% Power Driven to the Motors [W]
PowerDriven =2 * (MotorTorque * RPMSpeed/9.55 );

% Power Lost in Motor [W]
PowerDissM = PowerDriven * ((100-MotorEfficiency)/100);

% Power Lost in Motor Drive [W]
PowerDissMD = PowerDriven * ((100-DriveEfficiency)/100);

% Total Power Loss in Drive & Motor
TotalPowerDiss = PowerDissMD + PowerDissM;

% Total Power Out
PowerOut = PowerDriven - TotalPowerDiss;

% ---------------------------------------------%


end

== matlab function VehicleModel_V3/Optimised Speed Calculation ==
  data: remaining input; target output; u input
function  target=test(remaining,u)
    % Motor Parameters
    MotorEfficiency = 98.3;  % percent
    PeakTorque = 80;         %Nm
    MinimumDriveEfficiency = 94 ;     % percent

    % Wheel Parameters
    MotorDiameter = 0.38;        % meters
    TyreRimDiameter = 0.0762;    % meters


    %convert distance to meters
    remaining=remaining*1000;
    %create a 2d array of the times stores array as time then speed
    times=zeros(25,2);
    
    %create a 2d array of the driving power stores array as time then speed
    power=zeros(25,2);
    
    cost=zeros(25,2);

    r=1;
    %loop through range of speeds
    for i=12:36
        %%%%%Time to next checkpoint
        time=remaining/i;
        
        %%%%%%%power that is driving the wheels
        % Torque Driven to Motors
        MotorTorque = PeakTorque * u;
        % Total Diameter of Wheel
        WheelDiameter = MotorDiameter+TyreRimDiameter;
        % motor Speed m/s
        MSSpeed = i/3.6;
        % RPM
        RPMSpeed = 9.55 * (MSSpeed/(WheelDiameter/2));
        % rad/s
        WSpeed = (RPMSpeed/60) * (2*3.14159);
        % Motor Drive Efficiency at Motor Torque
        DriveEfficiency = MinimumDriveEfficiency + (WSpeed*0.1);
        % Power Driven to the Motors [W]
        PowerDriven =2 * (MotorTorque * RPMSpeed/9.55 );
        % Power Lost in Motor [W]
        PowerDissM = PowerDriven * ((100-MotorEfficiency)/100);
        % Power Lost in Motor Drive [W]
        PowerDissMD = PowerDriven * ((100-DriveEfficiency)/100);
        % Total Power Loss in Drive & Motor
        TotalPowerDiss = PowerDissMD + PowerDissM;
        % Total Power Out
        Pout = PowerDriven - TotalPowerDiss;
        
        
        
        cost(r,2)=i;
        cost(r,1)=(time/10) +Pout;
        
        
        r=r+1;
        
        
        
    end
    
    %%%
    %Perform bubble sort on the cost array to get column 1 in order
    %%%Will sort array so that the lowest cost is shown first then the
    %%%rest will be shown in ascending order
    % Traverse through all array elements
    for i=1:20
    % range(n) also work but outer loop will
    % repeat one time more than needed.
        % Last i elements are already in place
        for j=1:19
            % traverse the array from 0 to n-i-1
            % Swap if the element found is greater
            % than the next element
            if cost(j,1) > cost(j+1,1)
                temp1=cost(j,1);
                temp2=cost(j,2);
                cost(j,1)=cost(j+1,1);
                cost(j,2)=cost(j+1,2);
                cost(j+1,1) = temp1;
                cost(j+1,2) = temp2;
            end
        end
    end
    
    disp(cost);
    %the first item in the second column will be the ideal speed
    target=cost(1,2);
    
end

== matlab function VehicleModel_V3/Vehicle/MATLAB Function ==
  data: Speed input; Drag output; Volume parameter; drag_coeff parameter; front_area parameter
function Drag = fcn(Speed, Volume, drag_coeff, front_area)

%density is mass over volume.
density=800/Volume;

Drag=0.5*density*Speed^2*2*front_area*drag_coeff;

== matlab function VehicleModel_V3/Subsystem2/MATLAB Function ==
  data: V input; y output; I input; Vo input; Io input; D input
function y = inc(V, ... %Intial Voltage input
                 I, ... %Intial Current input
                 Vo, ... %Delayed Voltage input
                 Io, ... %Delayed Current input
                 D) %Delayed duty cycle input

m= 0.4; %Starting duty cycle 

dV= V-Vo; %Change in voltage

dI= I-Io; %Change in current

d=0.00005; %Duty cycle change

    if dV==0 %If the rate of change of voltage is zero

        if dI==0 %Check if the same applies to current

            m=D; %If then the starting duty cycle can be output

        else %If not assume the rate of change of voltage is greater than zero

            if dI>0

                m=D-d; %If the rate of change of current is greater than zero then reduce the duty cycle by a small margin
            else 

                m=D+d; %If the rate of change of current is less than zero then increase the duty cycle by a small margin

            end 

        end

    else 
        if dI/dV==-(I/V) %If the incremental inductace is equivalent to the negative instantaneous inductance

            m=D-d; %Then reduce the duty by a small margin 

        else 

            m=D+d;%Then increase the duty cycle by a small margin

        end
        
    end

y = D; % Output final value of duty cycle

== matlab function VehicleModel_V3/Subsystem2/MATLAB Function3 ==
  data: V input; y output; I input; Vo input; Io input; D input
function y = inc(V, ... %Intial Voltage input
                 I, ... %Intial Current input
                 Vo, ... %Delayed Voltage input
                 Io, ... %Delayed Current input
                 D) %Delayed duty cycle input

m= 0.4; %Starting duty cycle 

dV= V-Vo; %Change in voltage

dI= I-Io; %Change in current

d=0.00005; %Duty cycle change

    if dV==0 %If the rate of change of voltage is zero

        if dI==0 %Check if the same applies to current

            m=D; %If then the starting duty cycle can be output

        else %If not assume the rate of change of voltage is greater than zero

            if dI>0

                m=D-d; %If the rate of change of current is greater than zero then reduce the duty cycle by a small margin
            else 

                m=D+d; %If the rate of change of current is less than zero then increase the duty cycle by a small margin

            end 

        end

    else 
        if dI/dV==-(I/V) %If the incremental inductace is equivalent to the negative instantaneous inductance

            m=D-d; %Then reduce the duty by a small margin 

        else 

            m=D+d;%Then increase the duty cycle by a small margin

        end
        
    end

y = D; % Output final value of duty cycle

== matlab function VehicleModel_V3/Subsystem2/MATLAB Function4 ==
  data: V input; y output; I input; Vo input; Io input; D input
function y = inc(V, ... %Intial Voltage input
                 I, ... %Intial Current input
                 Vo, ... %Delayed Voltage input
                 Io, ... %Delayed Current input
                 D) %Delayed duty cycle input

m= 0.4; %Starting duty cycle 

dV= V-Vo; %Change in voltage

dI= I-Io; %Change in current

d=0.00005; %Duty cycle change

    if dV==0 %If the rate of change of voltage is zero

        if dI==0 %Check if the same applies to current

            m=D; %If then the starting duty cycle can be output

        else %If not assume the rate of change of voltage is greater than zero

            if dI>0

                m=D-d; %If the rate of change of current is greater than zero then reduce the duty cycle by a small margin
            else 

                m=D+d; %If the rate of change of current is less than zero then increase the duty cycle by a small margin

            end 

        end

    else 
        if dI/dV==-(I/V) %If the incremental inductace is equivalent to the negative instantaneous inductance

            m=D-d; %Then reduce the duty by a small margin 

        else 

            m=D+d;%Then increase the duty cycle by a small margin

        end
        
    end

y = D; % Output final value of duty cycle
